simulink model "lab_5_qpsk_viterbi_sqrt_equalizer"  (R2012b)
settings: Solver=ode45  SolverMode=SingleTasking  StartTime=0.0  StopTime=inf  RelTol=1e-3
values from neighbouring files (symbols this model uses):
  EbNodB = EbNoVec(n)    [a1.m]    (also in a2.m = 11; cawgn.m = (1/4) * Nvar + 5; lab_5_Pber.m = 13; lab_5_Propyskna_Zdatnist.m = 11)
  Fc = 2*pi*Rs    (= 43.9822971503)    [lab_5_parameters.m]
  Rb = Nvar    (= 24)    [lab_5_Propyskna_Zdatnist.m]    (also in lab_5_parameters.m = 14)
  Tb = 1/Rb    (= 0.0416666666667)    [lab_5_Propyskna_Zdatnist.m]    (also in lab_5_parameters.m = 0.0714285714286)
  Td = Ts/128    (= 0.00111607142857)    [lab_5_parameters.m]
  Ts = 1/Rs    (= 0.142857142857)    [lab_5_parameters.m]
undefined symbols (not defined in the file or in its folder): dfilt, figposition, Fs
libraries: commsink2 x6, dspsnks4 x6, commdigbbndpm3 x4, dspsrcs4 x4, dsparch4 x4, dspsigops x3, commcnvcod2 x2, commchan3 x1, commrandsrc2 x1, dspindex x1, commfilt2 x1
CloseFcn:
  | clear convSigsOut
settings Model: RequirementInfo=9  CovMetricSettings=d  ExtModeTrigMode=oneshot  ExtModeArmWhenConnect=off  Creator=mikem  LastModifiedBy=yuw
settings DataIOCC: LimitDataPoints=off  SaveOutput=off  SaveTime=off  SignalLoggingName=convSigsOut
settings OptimizationCC: BlockReduction=off  BooleanDataType=off  InitFltsAndDblsToZero=on
settings DebuggingCC: SaveWithParameterizedLinksMsg=none  SignalResolutionControl=TryResolveAllWithWarning  SolverPrmCheckMsg=none  MultiTaskDSMMsg=warning  MultiTaskCondExecSysMsg=none  IntegerOverflowMsg=none  StrictBusMsg=None
settings HardwareCC: TargetUnknown=on
settings RTWCC: IncludeERTFirstTime=on
settings GRTTargetCC: TargetFcnLib=ansi_tfl_tmw.mat  CombineOutputUpdateFcns=off  GRTInterface=on

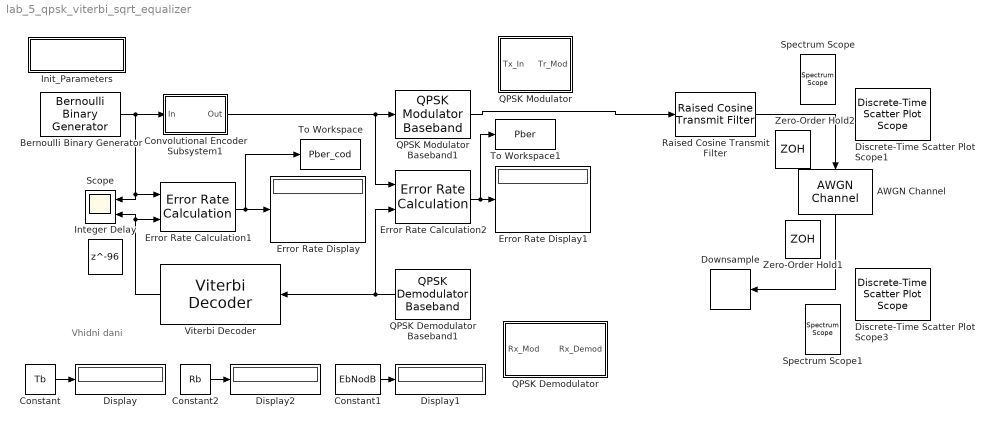
== system lab_5_qpsk_viterbi_sqrt_equalizer ==
  note: Vhidni dani
  AWGN Channel : commchan3/AWGN Channel  InputProcessing=Inherited (this choice will be removed - see release notes)  seed=54321  noiseMode="Signal to noise ratio  (Es/No)"  EbNodB=5  EsNodB=EbNodB+10*log10(1/2)  SNRdB=5  bitsPerSym=2  Ps=1  Tsym=1*Tb  variance=1
  Bernoulli Binary Generator : commrandsrc2/Bernoulli Binary Generator  P=0.5  seed=12345  Ts=Tb  frameBased=on  sampPerFrame=1  orient=off  outDataType=double
  Constant : Constant  Value=Tb
  Constant1 : Constant  Value=EbNodB
  Constant2 : Constant  Value=Rb
  Convolutional Encoder Subsystem1 : Subsystem
  Discrete-Time Scatter Plot Scope1 : commsink2/Discrete-Time Scatter Plot Scope  Tag=ScatterPlot  sampPerSymb=1  offsetEye=0  numTraces=40  numNewFrames=10  LineMarkers=.  LineColors=b  fading=on  render=on  AxisGrid=on  xMin=-1.5  xMax=1.5  yMin=-1.5  yMax=1.5  inphaseLabel=In-phase Amplitude  quadratureLabel=Quadrature Amplitude  openScopeAtSimStart=off  FrameNumber=off  FigPos=[360 138 560 560]  figTitle=Scatter Plot  numLinesMax=8  block_type_=scatter
  Discrete-Time Scatter Plot Scope3 : commsink2/Discrete-Time Scatter Plot Scope  Tag=ScatterPlot  sampPerSymb=1  offsetEye=0  numTraces=40  numNewFrames=10  LineMarkers=.  LineColors=b  fading=on  render=on  AxisGrid=on  xMin=-1.5  xMax=1.5  yMin=-1.5  yMax=1.5  inphaseLabel=In-phase Amplitude  quadratureLabel=Quadrature Amplitude  openScopeAtSimStart=off  FrameNumber=off  FigPos=[360 138 560 560]  figTitle=Scatter Plot  numLinesMax=8  block_type_=scatter
  Display : Display
  Display1 : Display
  Display2 : Display
  Downsample : dspsigops/Downsample  N=8  phase=0  InputProcessing=Inherited (this choice will be removed - see release notes)  RateOptions=Enforce single-rate processing  smode=Allow multirate  fmode=Maintain input frame rate  ic=0
  Error Rate Calculation1 : commsink2/Error Rate Calculation  N=96  st_delay=0  cp_mode=Entire frame  subframe=[]  PMode=Port  WsName=ErrorVec  RsMode2=off  stop=off  numErr=100  maxBits=1e7
  Error Rate Calculation2 : commsink2/Error Rate Calculation  N=0  st_delay=0  cp_mode=Entire frame  subframe=[]  PMode=Port  WsName=ErrorVec  RsMode2=off  stop=off  numErr=100  maxBits=1e6
  Error Rate Display : Display
  Error Rate Display1 : Display
  Init_Parameters : Subsystem
      settings: OpenFcn=lab_3_parameters
      mask Display: disp('lab_3_parameters')
  Integer Delay : Delay  DelayLength=96  InputProcessing=Inherited
  QPSK Demodulator Baseband1 : commdigbbndpm3/QPSK Demodulator Baseband  Ph=pi/4  Dec=Gray  OutType=Integer  DecType=Hard decision  VarSource=Dialog  Variance=1  outDtype1=Inherit via internal rule  outDtype2=Inherit via internal rule  derotateFactorWordLen=16
  QPSK Modulator Baseband1 : commdigbbndpm3/QPSK Modulator Baseband  InType=Integer  Enc=Gray  Ph=pi/4  outDtype=double  outWordLen=16  outUDDataType=sfix(16)  outFracLenMode=Best precision  outFracLen=15
  QPSK Demodulator : Subsystem
  QPSK Modulator : Subsystem
  Raised Cosine Transmit Filter : commfilt2/Raised Cosine Transmit Filter  filtType=Normal  D=3  R=0.5  sampMode=Mute  saveAsFlag=0  N=8  framing=Maintain input frame rate  InputProcessing=Columns as channels (frame based)  checkGain=Normalized  filterGain=1  checkCoeff=off  variableName=rcTxFilt  launchFVT=off  roundingMode=Floor  overflowMode=off
      link override Check Signal Attributes: Frame=Frame-based  Dimensions=Column vector (2-D) or scalar
      link override FIR Interpolation: framing=Maintain input frame rate
  Scope : Scope  NumInputPorts=2
      settings: YMin=-2~-2  YMax=2~2
  Spectrum Scope : dspsnks4/Spectrum Scope  ScopeProperties=on  Domain=Frequency  HorizSpan=1  UseBuffer=on  BufferSize=256  Overlap=0  TreatMby1Signals=M channels  inpFftLenInherit=off  FFTlength=128  numAvg=20  DisplayProperties=off  AxisGrid=on  Memory=off  FrameNumber=off  AxisLegend=off  AxisZoom=off  OpenScopeAtSimStart=off  OpenScopeImmediately=off  FigPos="figposition([7    12    39    27])"  AxisProperties=off  XUnits=Hertz  XRange=[-Fs/2...Fs/2]  XDisplay=0  InheritXIncr=on  XIncr=1.0  XLabel=Samples  XLimit=Auto  YUnits=dB  XMax=1  XMin=0  YLabel=Magnitude-squared, dB  LineProperties=off  LineColors=[1 0 0]  wintypeSpecScope=Hann  RsSpecScope=50  betaSpecScope=5  winsampSpecScope=Periodic  XAxisParamsVer=6.8  isFrameUpgraded=on
      settings: YMin=-50  YMax=10
  Spectrum Scope1 : dspsnks4/Spectrum Scope  ScopeProperties=on  Domain=Frequency  HorizSpan=1  UseBuffer=on  BufferSize=256  Overlap=0  TreatMby1Signals=M channels  inpFftLenInherit=off  FFTlength=128  numAvg=20  DisplayProperties=off  AxisGrid=on  Memory=off  FrameNumber=off  AxisLegend=off  AxisZoom=off  OpenScopeAtSimStart=off  OpenScopeImmediately=off  FigPos="figposition([49    12    39    27])"  AxisProperties=off  XUnits=Hertz  XRange=[-Fs/2...Fs/2]  XDisplay=0  InheritXIncr=on  XIncr=1.0  XLabel=Samples  XLimit=Auto  YUnits=dB  XMax=1  XMin=0  YLabel=Magnitude-squared, dB  LineProperties=off  LineColors=[1 0 0]  wintypeSpecScope=Hann  RsSpecScope=50  betaSpecScope=5  winsampSpecScope=Periodic  XAxisParamsVer=6.8  isFrameUpgraded=on
      settings: YMin=-10  YMax=10
  To Workspace : ToWorkspace  VariableName=Pber_cod  SampleTime=-1
      settings: MaxDataPoints=1
  To Workspace1 : ToWorkspace  VariableName=Pber  SampleTime=-1
      settings: MaxDataPoints=1
  Viterbi Decoder : commcnvcod2/Viterbi Decoder  trellis=poly2trellis(7, [171 133])  isPunctured=off  punctureVector=[1; 1; 0; 1; 0; 1]  erasures=off  dectype=Hard decision  runSigValErrCheck=off  nsdecb=4  smWordLength=16  tbdepth=96  opmode=Continuous  reset=off  outDataType=double  delayedResetAction=off
  Zero-Order Hold1 : ZeroOrderHold  SampleTime=Td
  Zero-Order Hold2 : ZeroOrderHold  SampleTime=Td
  wires:
  Error Rate Calculation1/1 -> To Workspace/1, Error Rate Display/1
  Convolutional Encoder Subsystem1/1(Out) -> QPSK Modulator Baseband1/1, Error Rate Calculation2/1
  QPSK Demodulator Baseband1/1 -> Viterbi Decoder/1, Error Rate Calculation2/2
  Bernoulli Binary Generator/1 -> Error Rate Calculation1/1, Scope/1, Convolutional Encoder Subsystem1/1(In)
  Constant/1 -> Display/1
  Constant1/1 -> Display1/1
  Constant2/1 -> Display2/1
  Error Rate Calculation2/1 -> Error Rate Display1/1, To Workspace1/1
  Viterbi Decoder/1 -> Scope/2, Error Rate Calculation1/2
  Raised Cosine Transmit Filter/1 -> AWGN Channel/1
  QPSK Modulator Baseband1/1 -> Raised Cosine Transmit Filter/1
  AWGN Channel/1 -> Downsample/1

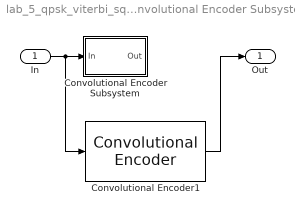
== system lab_5_qpsk_viterbi_sqrt_equalizer/Convolutional Encoder Subsystem1 ==
  In : Inport
  Convolutional Encoder Subsystem : Subsystem
  Convolutional Encoder1 : commcnvcod2/Convolutional Encoder  trellis=poly2trellis(7, [171 133])  opMode=Continuous  DelayedResetAction=off  hasIniStPort=off  hasFinStPort=off  usePuncVector=off  punctureVector=[1; 1; 0; 1; 0; 1]  reset=Unused parameter value
  Out : Outport
  wires:
  In/1 -> Convolutional Encoder Subsystem/1(In), Convolutional Encoder1/1
  Convolutional Encoder1/1 -> Out/1

== system lab_5_qpsk_viterbi_sqrt_equalizer/Init_Parameters ==

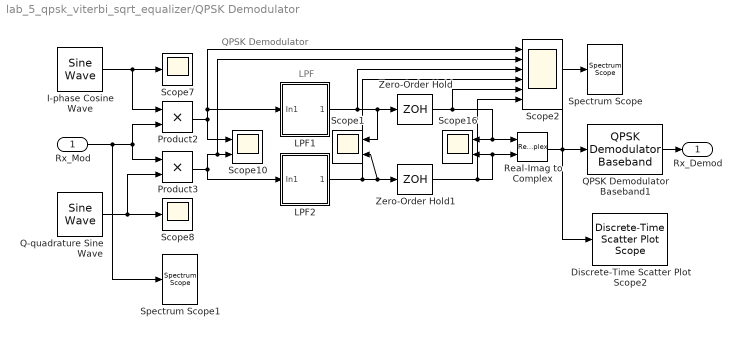
== system lab_5_qpsk_viterbi_sqrt_equalizer/QPSK Demodulator ==
  note: QPSK Demodulator
  note: LPF
  Rx_Mod : Inport
  Discrete-Time Scatter Plot Scope2 : commsink2/Discrete-Time Scatter Plot Scope  Tag=ScatterPlot  sampPerSymb=1  offsetEye=0  numTraces=40  numNewFrames=10  LineMarkers=.  LineColors=b  fading=on  render=on  AxisGrid=on  xMin=-1.5  xMax=1.5  yMin=-1.5  yMax=1.5  inphaseLabel=In-phase Amplitude  quadratureLabel=Quadrature Amplitude  openScopeAtSimStart=on  FrameNumber=off  FigPos=[360 138 560 560]  figTitle=Scatter Plot  numLinesMax=8  block_type_=scatter
  I-phase Cosine Wave : dspsrcs4/Sine Wave  Amplitude=sqrt(2)  Frequency=Fc  Phase=pi/2  SampleMode=Discrete  OutComplex=Real  CompMethod=Trigonometric fcn  TableSize=Speed  SampleTime=Td  SamplesPerFrame=1  ResetState=Restart at time zero  dataType=double  wordLen=16  udDataType=sfix(16)  fracBitsMode=Best precision  numFracBits=15  OutDataTypeStr=double  LastOutDataTypeStr=double
  LPF1 : Subsystem
  LPF2 : Subsystem
  Product2 : Product  RndMeth=Zero
  Product3 : Product  RndMeth=Zero
  Q-quadrature Sine Wave : dspsrcs4/Sine Wave  Amplitude=sqrt(2)  Frequency=Fc  Phase=pi  SampleMode=Discrete  OutComplex=Real  CompMethod=Trigonometric fcn  TableSize=Speed  SampleTime=Td  SamplesPerFrame=1  ResetState=Restart at time zero  dataType=double  wordLen=16  udDataType=sfix(16)  fracBitsMode=Best precision  numFracBits=15  OutDataTypeStr=double  LastOutDataTypeStr=double
  QPSK Demodulator Baseband1 : commdigbbndpm3/QPSK Demodulator Baseband  Ph=pi/4  Dec=Gray  OutType=Integer  DecType=Hard decision  VarSource=Dialog  Variance=1  outDtype1=Inherit via internal rule  outDtype2=Inherit via internal rule  derotateFactorWordLen=16
  Real-Imag to Complex : RealImagToComplex
  Scope1 : Scope  NumInputPorts=2
      settings: YMin=-5~-5  YMax=5~5  SaveName=ScopeData4
  Scope10 : Scope  NumInputPorts=2
      settings: YMin=-5~-5  YMax=5~5  SaveName=ScopeData10
  Scope16 : Scope  NumInputPorts=2
      settings: YMin=-5~-5  YMax=5~5
  Scope2 : Scope  NumInputPorts=6
      settings: YMin=-5~-5~-5~-5~-5~-5  YMax=5~5~5~5~5~5  SaveName=ScopeData12
  Scope7 : Scope
      settings: SaveName=ScopeData7
  Scope8 : Scope
      settings: SaveName=ScopeData8
  Spectrum Scope : dspsnks4/Spectrum Scope  ScopeProperties=on  Domain=Frequency  HorizSpan=1  UseBuffer=on  BufferSize=256  Overlap=0  TreatMby1Signals=M channels  inpFftLenInherit=off  FFTlength=128  numAvg=20  DisplayProperties=off  AxisGrid=on  Memory=off  FrameNumber=off  AxisLegend=off  AxisZoom=off  OpenScopeAtSimStart=off  OpenScopeImmediately=off  FigPos="figposition([49    12    39    27])"  AxisProperties=off  XUnits=Hertz  XRange=[-Fs/2...Fs/2]  XDisplay=0  InheritXIncr=on  XIncr=1.0  XLabel=Samples  XLimit=Auto  YUnits=dB  XMax=1  XMin=0  YLabel=Magnitude-squared, dB  LineProperties=off  LineColors=[1 0 0]  wintypeSpecScope=Hann  RsSpecScope=50  betaSpecScope=5  winsampSpecScope=Periodic  XAxisParamsVer=6.8  isFrameUpgraded=on
      settings: YMin=-10  YMax=10
  Spectrum Scope1 : dspsnks4/Spectrum Scope  ScopeProperties=on  Domain=Frequency  HorizSpan=1  UseBuffer=on  BufferSize=256  Overlap=0  TreatMby1Signals=M channels  inpFftLenInherit=off  FFTlength=128  numAvg=20  DisplayProperties=off  AxisGrid=on  Memory=off  FrameNumber=off  AxisLegend=off  AxisZoom=off  OpenScopeAtSimStart=on  OpenScopeImmediately=off  FigPos="figposition([49    12    39    27])"  AxisProperties=off  XUnits=Hertz  XRange=[-Fs/2...Fs/2]  XDisplay=0  InheritXIncr=on  XIncr=1.0  XLabel=Samples  XLimit=Auto  YUnits=dB  XMax=1  XMin=0  YLabel=Magnitude-squared, dB  LineProperties=off  LineColors=[1 0 0]  wintypeSpecScope=Hann  RsSpecScope=50  betaSpecScope=5  winsampSpecScope=Periodic  XAxisParamsVer=6.8  isFrameUpgraded=on
      settings: YMin=-10  YMax=10
  Zero-Order Hold : ZeroOrderHold  SampleTime=Ts
  Zero-Order Hold1 : ZeroOrderHold  SampleTime=Ts
  Rx_Demod : Outport
  wires:
  Zero-Order Hold1/1 -> Scope2/6, Scope16/2, Real-Imag to Complex/2
  Zero-Order Hold/1 -> Scope2/5, Scope16/1, Real-Imag to Complex/1
  LPF2/1(Out1) -> Scope2/4, Scope1/2, Zero-Order Hold1/1
  Product2/1 -> Scope2/1, LPF1/1(In1), Scope10/1
  Product3/1 -> Scope2/2, Scope10/2, LPF2/1(In1)
  LPF1/1(Out1) -> Scope2/3, Scope1/1, Zero-Order Hold/1
  QPSK Demodulator Baseband1/1 -> Rx_Demod/1
  Rx_Mod/1 -> Spectrum Scope1/1, Product3/1, Product2/2
  Real-Imag to Complex/1 -> QPSK Demodulator Baseband1/1, Discrete-Time Scatter Plot Scope2/1, Spectrum Scope/1
  Q-quadrature Sine Wave/1 -> Product3/2, Scope8/1
  I-phase Cosine Wave/1 -> Product2/1, Scope7/1

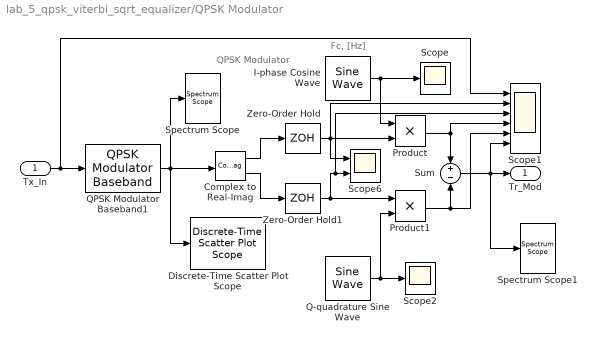
== system lab_5_qpsk_viterbi_sqrt_equalizer/QPSK Modulator ==
  note: Fc, [Hz]
  note: QPSK Modulator
  Tx_In : Inport
  Complex to Real-Imag : ComplexToRealImag
  Discrete-Time Scatter Plot Scope : commsink2/Discrete-Time Scatter Plot Scope  Tag=ScatterPlot  sampPerSymb=1  offsetEye=0  numTraces=40  numNewFrames=10  LineMarkers=.  LineColors=b  fading=on  render=on  AxisGrid=on  xMin=-1.5  xMax=1.5  yMin=-1.5  yMax=1.5  inphaseLabel=In-phase Amplitude  quadratureLabel=Quadrature Amplitude  openScopeAtSimStart=on  FrameNumber=off  FigPos=[360 138 560 560]  figTitle=Scatter Plot  numLinesMax=8  block_type_=scatter
  I-phase Cosine Wave : dspsrcs4/Sine Wave  Amplitude=sqrt(2)  Frequency=Fc  Phase=pi/2  SampleMode=Discrete  OutComplex=Real  CompMethod=Trigonometric fcn  TableSize=Speed  SampleTime=Td  SamplesPerFrame=1  ResetState=Restart at time zero  dataType=double  wordLen=16  udDataType=sfix(16)  fracBitsMode=Best precision  numFracBits=15  OutDataTypeStr=double  LastOutDataTypeStr=double
  Product : Product  RndMeth=Zero
  Product1 : Product  RndMeth=Zero
  Q-quadrature Sine Wave : dspsrcs4/Sine Wave  Amplitude=1  Frequency=Fc  Phase=0  SampleMode=Discrete  OutComplex=Real  CompMethod=Trigonometric fcn  TableSize=Speed  SampleTime=Td  SamplesPerFrame=1  ResetState=Restart at time zero  dataType=double  wordLen=16  udDataType=sfix(16)  fracBitsMode=Best precision  numFracBits=15  OutDataTypeStr=double  LastOutDataTypeStr=double
  QPSK Modulator Baseband1 : commdigbbndpm3/QPSK Modulator Baseband  InType=Integer  Enc=Gray  Ph=pi/4  outDtype=double  outWordLen=16  outUDDataType=sfix(16)  outFracLenMode=Best precision  outFracLen=15
  Scope : Scope
      settings: SaveName=ScopeData2
  Scope1 : Scope  NumInputPorts=6
      settings: TimeRange=5  YMin=-5~-5~-5~-5~-5~-5  YMax=5~5~5~5~5~5
  Scope2 : Scope
      settings: SaveName=ScopeData3
  Scope6 : Scope  NumInputPorts=2
      settings: YMin=-5~-5  YMax=5~5  SaveName=ScopeData6
  Spectrum Scope : dspsnks4/Spectrum Scope  ScopeProperties=on  Domain=Frequency  HorizSpan=1  UseBuffer=on  BufferSize=256  Overlap=0  TreatMby1Signals=M channels  inpFftLenInherit=off  FFTlength=128  numAvg=20  DisplayProperties=off  AxisGrid=on  Memory=off  FrameNumber=off  AxisLegend=off  AxisZoom=off  OpenScopeAtSimStart=off  OpenScopeImmediately=off  FigPos="figposition([49    12    39    27])"  AxisProperties=off  XUnits=Hertz  XRange=[-Fs/2...Fs/2]  XDisplay=0  InheritXIncr=on  XIncr=1.0  XLabel=Samples  XLimit=Auto  YUnits=dB  XMax=1  XMin=0  YLabel=Magnitude-squared, dB  LineProperties=off  LineColors=[1 0 0]  wintypeSpecScope=Hann  RsSpecScope=50  betaSpecScope=5  winsampSpecScope=Periodic  XAxisParamsVer=6.8  isFrameUpgraded=on
      settings: YMin=-10  YMax=10
  Spectrum Scope1 : dspsnks4/Spectrum Scope  ScopeProperties=on  Domain=Frequency  HorizSpan=1  UseBuffer=on  BufferSize=256  Overlap=0  TreatMby1Signals=M channels  inpFftLenInherit=off  FFTlength=128  numAvg=20  DisplayProperties=off  AxisGrid=on  Memory=off  FrameNumber=off  AxisLegend=off  AxisZoom=off  OpenScopeAtSimStart=on  OpenScopeImmediately=off  FigPos="figposition([49    12    39    27])"  AxisProperties=off  XUnits=Hertz  XRange=[-Fs/2...Fs/2]  XDisplay=0  InheritXIncr=on  XIncr=1.0  XLabel=Samples  XLimit=Auto  YUnits=dB  XMax=1  XMin=0  YLabel=Magnitude-squared, dB  LineProperties=off  LineColors=[1 0 0]  wintypeSpecScope=Hann  RsSpecScope=50  betaSpecScope=5  winsampSpecScope=Periodic  XAxisParamsVer=6.8  isFrameUpgraded=on
      settings: YMin=-10  YMax=10
  Sum : Sum  Inputs=+-
  Zero-Order Hold : ZeroOrderHold  SampleTime=Ts
  Zero-Order Hold1 : ZeroOrderHold  SampleTime=Ts
  Tr_Mod : Outport
  wires:
  Zero-Order Hold/1 -> Scope1/2, Scope6/1, Product/2
  Q-quadrature Sine Wave/1 -> Scope2/1, Product1/2
  I-phase Cosine Wave/1 -> Scope/1, Product/1
  Zero-Order Hold1/1 -> Scope1/3, Scope6/2, Product1/1
  Complex to Real-Imag/1 -> Zero-Order Hold/1
  Complex to Real-Imag/2 -> Zero-Order Hold1/1
  Tx_In/1 -> QPSK Modulator Baseband1/1, Scope1/1
  Sum/1 -> Scope1/6, Spectrum Scope1/1, Tr_Mod/1
  Product/1 -> Scope1/4, Sum/1
  QPSK Modulator Baseband1/1 -> Discrete-Time Scatter Plot Scope/1, Spectrum Scope/1, Complex to Real-Imag/1
  Product1/1 -> Scope1/5, Sum/2

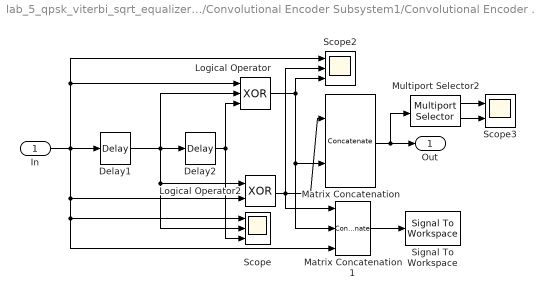
== system lab_5_qpsk_viterbi_sqrt_equalizer/Convolutional Encoder Subsystem1/Convolutional Encoder Subsystem ==
  In : Inport
  Delay1 : dspsigops/Delay  InputProcessing=Inherited (this choice will be removed - see release notes)  dly_unit=Samples  delay=1  ic_detail=off  dif_ic_for_ch=off  dif_ic_for_dly=off  ic=0  reset_popup=None
  Delay2 : dspsigops/Delay  InputProcessing=Inherited (this choice will be removed - see release notes)  dly_unit=Samples  delay=1  ic_detail=off  dif_ic_for_ch=off  dif_ic_for_dly=off  ic=0  reset_popup=None
  Logical Operator : Logic  Operator=XOR  Inputs=3  AllPortsSameDT=off
  Logical Operator2 : Logic  Operator=XOR  AllPortsSameDT=off
  Matrix Concatenation : Concatenate  Mode=Multidimensional array
  Matrix Concatenation1 : Concatenate  NumInputs=3  Mode=Multidimensional array  ConcatenateDimension=2
  Multiport Selector2 : dspindex/Multiport Selector  rowsOrCols=Rows  idxCellArray={1 2}  idxErrMode=Clip Index
  Scope : Scope  NumInputPorts=3
      settings: YMin=-5~-5~-5  YMax=5~5~5
  Scope2 : Scope  NumInputPorts=3
      settings: YMin=-5~-5~-5  YMax=5~5~5  SaveName=ScopeData2
  Scope3 : Scope  NumInputPorts=2
      settings: YMin=-5~-5  YMax=5~5  SaveName=ScopeData3
  Signal To Workspace : SignalToWorkspace  VariableName=In_Cod
      settings: CopyFcn=dspblkcopystw(gcbh);
  Out : Outport
  wires:
  Delay2/1 -> Logical Operator/3, Scope/3
  Delay1/1 -> Delay2/1, Logical Operator/2, Scope/2, Logical Operator2/1
  Multiport Selector2/1 -> Scope3/1
  Multiport Selector2/2 -> Scope3/2
  Logical Operator/1 -> Scope2/3, Matrix Concatenation/2, Matrix Concatenation1/2
  Logical Operator2/1 -> Scope2/2, Matrix Concatenation/1, Matrix Concatenation1/1
  In/1 -> Delay1/1, Logical Operator2/2, Scope/1, Matrix Concatenation1/3, Logical Operator/1, Scope2/1
  Matrix Concatenation/1 -> Out/1, Multiport Selector2/1
  Matrix Concatenation1/1 -> Signal To Workspace/1

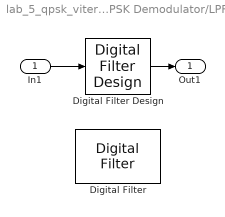
== system lab_5_qpsk_viterbi_sqrt_equalizer/QPSK Demodulator/LPF1 ==
  In1 : Inport
  Digital Filter Design : dsparch4/Digital Filter Design  mwdsp_browser_bugfix_var=off
  Digital Filter : dsparch4/Digital Filter  TypePopup=FIR (all zeros)  IIRFiltStruct=Direct form II transposed  AllPoleFiltStruct=Direct form  FIRFiltStruct=Direct form  CoeffSource=Specify via dialog  NumCoeffs=[1 2]  DenCoeffs=[1 0.1]  BiQuadCoeffs=[1 0.3 0.4 1 0.1 0.2]  LatticeCoeffs=[0.2 0.4]  denIgnore=on  FiltPerSampPopup=One filter per frame  IC=0  ICnum=0  ICden=0  roundingMode=Floor  overflowMode=off  ScaleValues=1  scaleValueFracLength=14  stageInFracLength=15  stageOutFracLength=15  FilterSource=Specify via dialog  dfiltObjectName=dfilt.dffir([1 2 1])  InputProcessing=Inherited (this choice will be removed - see release notes)
  Out1 : Outport
  wires:
  Digital Filter Design/1 -> Out1/1
  In1/1 -> Digital Filter Design/1

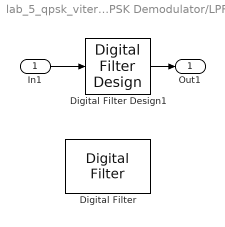
== system lab_5_qpsk_viterbi_sqrt_equalizer/QPSK Demodulator/LPF2 ==
  In1 : Inport
  Digital Filter Design1 : dsparch4/Digital Filter Design  mwdsp_browser_bugfix_var=off
  Digital Filter : dsparch4/Digital Filter  TypePopup=IIR (poles & zeros)  IIRFiltStruct=Direct form II transposed  AllPoleFiltStruct=Direct form  FIRFiltStruct=Direct form  CoeffSource=Specify via dialog  NumCoeffs=[1 2]  DenCoeffs=[1 0.1]  BiQuadCoeffs=[1 0.3 0.4 1 0.1 0.2]  LatticeCoeffs=[0.2 0.4]  denIgnore=on  FiltPerSampPopup=One filter per frame  IC=0  ICnum=0  ICden=0  roundingMode=Floor  overflowMode=off  ScaleValues=1  scaleValueFracLength=14  stageInFracLength=15  stageOutFracLength=15  FilterSource=Specify via dialog  dfiltObjectName=dfilt.dffir([1 2 1])  InputProcessing=Inherited (this choice will be removed - see release notes)
  Out1 : Outport
  wires:
  Digital Filter Design1/1 -> Out1/1
  In1/1 -> Digital Filter Design1/1
